simulink model "Model_V5"  (R2024b)
settings: Solver=VariableStepAuto  StartTime=0.0  StopTime=3600*12  RelTol=1e-3
undefined symbols (not defined in the file): PropsSI
libraries: fl_lib x569, SimscapeFluids_lib x61, nesl_utility x27
(part 2 of 7)

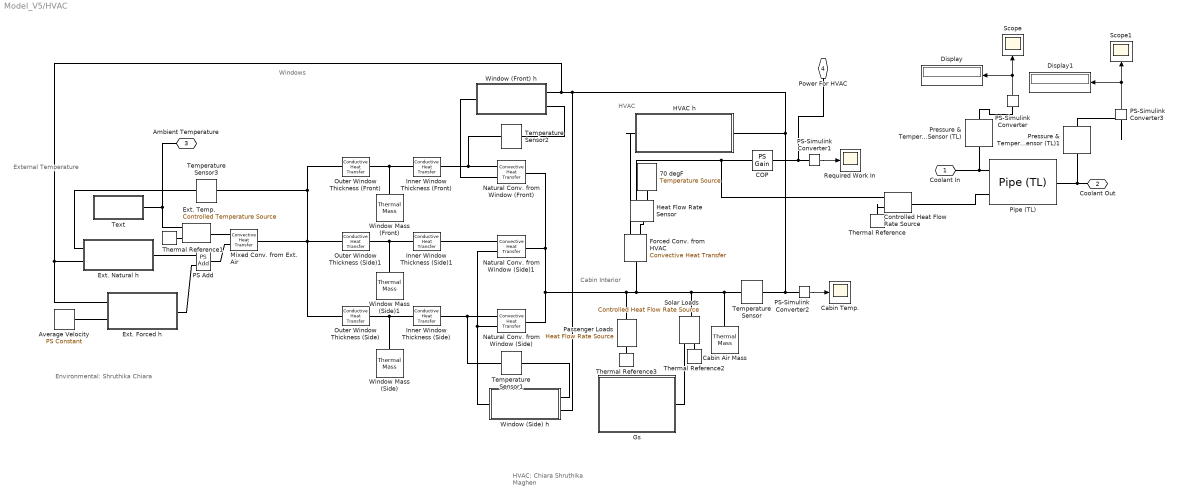
== system Model_V5/HVAC ==
  note: HVAC:
      | Chiara
      | Shruthika
      | Maghen
  note: Environmental:
      | Shruthika
      | Chiara
  note: Cabin Interior
  note: HVAC
  note: External Temperature
  note: Windows
  70 degF : fl_lib/Thermal/Thermal Sources/Temperature Source  temperature=70 degF
  Average Velocity : fl_lib/Physical Signals/Sources/PS Constant  constant=48 mi/hr
  COP : fl_lib/Physical Signals/Functions/PS Gain  gain=1/2
  Cabin Air Mass : fl_lib/Thermal/Thermal Elements/Thermal Mass  mass_type=foundation.enum.constant_variable.constant  mass=9.4009 kg  sp_heat=1005 J/(K*kg)  mass_min=1e-6 kg  num_ports=foundation.enum.numPorts2.one  m_specify=off  m_priority=High  m=1 kg  m_nominal_specify=off  m_nominal_value=1  m_nominal_unit=kg  T_specify=on  T_priority=Low  T=70 degF  T_nominal_specify=off  T_nominal_value=1  T_nominal_unit=K  Q_specify=off  Q_priority=None  Q=0 W  Q_nominal_specify=off  Q_nominal_value=1  Q_nominal_unit=W
  Cabin Temp. : Scope
  Controlled Heat Flow Rate Source : fl_lib/Thermal/Thermal Sources/Controlled Heat Flow Rate Source
  Display : Display
  Display1 : Display
  Ext. Forced h : Subsystem
  Ext. Natural h : Subsystem
  Ext. Temp. : fl_lib/Thermal/Thermal Sources/Controlled Temperature Source
  Forced Conv. from HVAC : fl_lib/Thermal/Thermal Elements/Convective Heat Transfer  thermal_type=foundation.enum.constant_variable.variable  area=19.0332 m^2  heat_tr_coeff=24.15 W/(K*m^2)  min_heat_tr_coeff=1e-3 W/(K*m^2)  T_specify=off  T_priority=None  T=0 K  T_nominal_specify=off  T_nominal_value=1  T_nominal_unit=K  Q_specify=off  Q_priority=None  Q=0 W  Q_nominal_specify=off  Q_nominal_value=1  Q_nominal_unit=W
      settings: InternalSimscapePortConfiguration="{\"Bottom\":[],\"Left\":[{\"id\":\"A\",\"label\":\"A\",\"type\":\"foundation.thermal.thermal\"},{\"id\":\"var_heat_tr_coeff\",\"label\":\"K\",\"type\":\"input\"}],\"Right\":[{\"id\":\"B\",\"label\":\"B\",\"type\":\"foundation.thermal.thermal\"}],\"Top\":[]}"
  Gs : Subsystem
  HVAC h : Subsystem
  Heat Flow Rate Sensor : fl_lib/Thermal/Thermal Sensors/Heat Flow Rate Sensor
  Inner Window Thickness (Front) : fl_lib/Thermal/Thermal Elements/Conductive Heat Transfer  thermal_type=foundation.enum.ConstantVariableTabulated.Constant  wall_geometry=foundation.enum.ConductionWallGeometry.Planar  area=40*55 in^2  thickness=0.25/2 in  d_in=0.05 m  d_out=0.1 m  L=1 m  th_cond_min=10 W/(K*m)  th_cond=1.05 W/(K*m)  th_cond_TLU=[413, 401, 392, 383, 371, 357, 342] W/(K*m)  temp_TLU=[200, 273, 400, 600, 800, 1000, 1200] K  T_specify=off  T_priority=None  T=0 K  T_nominal_specify=off  T_nominal_value=1  T_nominal_unit=K  Q_specify=off  Q_priority=None  Q=0 W  Q_nominal_specify=off  Q_nominal_value=1  Q_nominal_unit=W
  Inner Window Thickness (Side) : fl_lib/Thermal/Thermal Elements/Conductive Heat Transfer  thermal_type=foundation.enum.ConstantVariableTabulated.Constant  wall_geometry=foundation.enum.ConductionWallGeometry.Planar  area=40*40 in^2  thickness=0.25/2 in  d_in=0.05 m  d_out=0.1 m  L=1 m  th_cond_min=10 W/(K*m)  th_cond=1.05 W/(K*m)  th_cond_TLU=[413, 401, 392, 383, 371, 357, 342] W/(K*m)  temp_TLU=[200, 273, 400, 600, 800, 1000, 1200] K  T_specify=off  T_priority=None  T=0 K  T_nominal_specify=off  T_nominal_value=1  T_nominal_unit=K  Q_specify=off  Q_priority=None  Q=0 W  Q_nominal_specify=off  Q_nominal_value=1  Q_nominal_unit=W
  Inner Window Thickness (Side)1 : fl_lib/Thermal/Thermal Elements/Conductive Heat Transfer  thermal_type=foundation.enum.ConstantVariableTabulated.Constant  wall_geometry=foundation.enum.ConductionWallGeometry.Planar  area=40*40 in^2  thickness=0.25/2 in  d_in=0.05 m  d_out=0.1 m  L=1 m  th_cond_min=10 W/(K*m)  th_cond=1.05 W/(K*m)  th_cond_TLU=[413, 401, 392, 383, 371, 357, 342] W/(K*m)  temp_TLU=[200, 273, 400, 600, 800, 1000, 1200] K  T_specify=off  T_priority=None  T=0 K  T_nominal_specify=off  T_nominal_value=1  T_nominal_unit=K  Q_specify=off  Q_priority=None  Q=0 W  Q_nominal_specify=off  Q_nominal_value=1  Q_nominal_unit=W
  Mixed Conv. from Ext. Air : fl_lib/Thermal/Thermal Elements/Convective Heat Transfer  thermal_type=foundation.enum.constant_variable.variable  area=1e-4 m^2  heat_tr_coeff=20 W/(K*m^2)  min_heat_tr_coeff=1e-3 W/(K*m^2)  T_specify=off  T_priority=None  T=0 K  T_nominal_specify=off  T_nominal_value=1  T_nominal_unit=K  Q_specify=off  Q_priority=None  Q=0 W  Q_nominal_specify=off  Q_nominal_value=1  Q_nominal_unit=W
      settings: InternalSimscapePortConfiguration="{\"Bottom\":[],\"Left\":[{\"id\":\"A\",\"label\":\"A\",\"type\":\"foundation.thermal.thermal\"},{\"id\":\"var_heat_tr_coeff\",\"label\":\"K\",\"type\":\"input\"}],\"Right\":[{\"id\":\"B\",\"label\":\"B\",\"type\":\"foundation.thermal.thermal\"}],\"Top\":[]}"
  Natural Conv. from Window (Front) : fl_lib/Thermal/Thermal Elements/Convective Heat Transfer  thermal_type=foundation.enum.constant_variable.variable  area=1e-4 m^2  heat_tr_coeff=20 W/(K*m^2)  min_heat_tr_coeff=1e-3 W/(K*m^2)  T_specify=off  T_priority=None  T=0 K  T_nominal_specify=off  T_nominal_value=1  T_nominal_unit=K  Q_specify=off  Q_priority=None  Q=0 W  Q_nominal_specify=off  Q_nominal_value=1  Q_nominal_unit=W
      settings: InternalSimscapePortConfiguration="{\"Bottom\":[],\"Left\":[{\"id\":\"A\",\"label\":\"A\",\"type\":\"foundation.thermal.thermal\"},{\"id\":\"var_heat_tr_coeff\",\"label\":\"K\",\"type\":\"input\"}],\"Right\":[{\"id\":\"B\",\"label\":\"B\",\"type\":\"foundation.thermal.thermal\"}],\"Top\":[]}"
  Natural Conv. from Window (Side) : fl_lib/Thermal/Thermal Elements/Convective Heat Transfer  thermal_type=foundation.enum.constant_variable.variable  area=1e-4 m^2  heat_tr_coeff=20 W/(K*m^2)  min_heat_tr_coeff=1e-3 W/(K*m^2)  T_specify=off  T_priority=None  T=0 K  T_nominal_specify=off  T_nominal_value=1  T_nominal_unit=K  Q_specify=off  Q_priority=None  Q=0 W  Q_nominal_specify=off  Q_nominal_value=1  Q_nominal_unit=W
      settings: InternalSimscapePortConfiguration="{\"Bottom\":[],\"Left\":[{\"id\":\"A\",\"label\":\"A\",\"type\":\"foundation.thermal.thermal\"},{\"id\":\"var_heat_tr_coeff\",\"label\":\"K\",\"type\":\"input\"}],\"Right\":[{\"id\":\"B\",\"label\":\"B\",\"type\":\"foundation.thermal.thermal\"}],\"Top\":[]}"
  Natural Conv. from Window (Side)1 : fl_lib/Thermal/Thermal Elements/Convective Heat Transfer  thermal_type=foundation.enum.constant_variable.variable  area=1e-4 m^2  heat_tr_coeff=20 W/(K*m^2)  min_heat_tr_coeff=1e-3 W/(K*m^2)  T_specify=off  T_priority=None  T=0 K  T_nominal_specify=off  T_nominal_value=1  T_nominal_unit=K  Q_specify=off  Q_priority=None  Q=0 W  Q_nominal_specify=off  Q_nominal_value=1  Q_nominal_unit=W
      settings: InternalSimscapePortConfiguration="{\"Bottom\":[],\"Left\":[{\"id\":\"A\",\"label\":\"A\",\"type\":\"foundation.thermal.thermal\"},{\"id\":\"var_heat_tr_coeff\",\"label\":\"K\",\"type\":\"input\"}],\"Right\":[{\"id\":\"B\",\"label\":\"B\",\"type\":\"foundation.thermal.thermal\"}],\"Top\":[]}"
  Outer Window Thickness (Front) : fl_lib/Thermal/Thermal Elements/Conductive Heat Transfer  thermal_type=foundation.enum.ConstantVariableTabulated.Constant  wall_geometry=foundation.enum.ConductionWallGeometry.Planar  area=40*55 in^2  thickness=0.25/2 m  d_in=0.05 m  d_out=0.1 m  L=1 m  th_cond_min=10 W/(K*m)  th_cond=1.05 W/(K*m)  th_cond_TLU=[413, 401, 392, 383, 371, 357, 342] W/(K*m)  temp_TLU=[200, 273, 400, 600, 800, 1000, 1200] K  T_specify=off  T_priority=None  T=0 K  T_nominal_specify=off  T_nominal_value=1  T_nominal_unit=K  Q_specify=off  Q_priority=None  Q=0 W  Q_nominal_specify=off  Q_nominal_value=1  Q_nominal_unit=W
  Outer Window Thickness (Side) : fl_lib/Thermal/Thermal Elements/Conductive Heat Transfer  thermal_type=foundation.enum.ConstantVariableTabulated.Constant  wall_geometry=foundation.enum.ConductionWallGeometry.Planar  area=40*40 in^2  thickness=0.25/2 m  d_in=0.05 m  d_out=0.1 m  L=1 m  th_cond_min=10 W/(K*m)  th_cond=1.05 W/(K*m)  th_cond_TLU=[413, 401, 392, 383, 371, 357, 342] W/(K*m)  temp_TLU=[200, 273, 400, 600, 800, 1000, 1200] K  T_specify=off  T_priority=None  T=0 K  T_nominal_specify=off  T_nominal_value=1  T_nominal_unit=K  Q_specify=off  Q_priority=None  Q=0 W  Q_nominal_specify=off  Q_nominal_value=1  Q_nominal_unit=W
  Outer Window Thickness (Side)1 : fl_lib/Thermal/Thermal Elements/Conductive Heat Transfer  thermal_type=foundation.enum.ConstantVariableTabulated.Constant  wall_geometry=foundation.enum.ConductionWallGeometry.Planar  area=40*40 in^2  thickness=0.25/2 m  d_in=0.05 m  d_out=0.1 m  L=1 m  th_cond_min=10 W/(K*m)  th_cond=1.05 W/(K*m)  th_cond_TLU=[413, 401, 392, 383, 371, 357, 342] W/(K*m)  temp_TLU=[200, 273, 400, 600, 800, 1000, 1200] K  T_specify=off  T_priority=None  T=0 K  T_nominal_specify=off  T_nominal_value=1  T_nominal_unit=K  Q_specify=off  Q_priority=None  Q=0 W  Q_nominal_specify=off  Q_nominal_value=1  Q_nominal_unit=W
  PS Add : fl_lib/Physical Signals/Functions/PS Add
  PS-Simulink Converter : nesl_utility/PS-Simulink Converter  PhysicalDomain=network_engine_domain  SubClassName=ps_output  LeftPortType=input  RightPortType=output  PseudoPeriodic=off  Frequencies=[]  VectorFormat=inherit  Unit=degF  AffineConversion=on
  PS-Simulink Converter1 : nesl_utility/PS-Simulink Converter  PhysicalDomain=network_engine_domain  SubClassName=ps_output  LeftPortType=input  RightPortType=output  PseudoPeriodic=off  Frequencies=[]  VectorFormat=inherit  Unit=inherit  AffineConversion=off
  PS-Simulink Converter2 : nesl_utility/PS-Simulink Converter  PhysicalDomain=network_engine_domain  SubClassName=ps_output  LeftPortType=input  RightPortType=output  PseudoPeriodic=off  Frequencies=[]  VectorFormat=inherit  Unit=degF  AffineConversion=on
  PS-Simulink Converter3 : nesl_utility/PS-Simulink Converter  PhysicalDomain=network_engine_domain  SubClassName=ps_output  LeftPortType=input  RightPortType=output  PseudoPeriodic=off  Frequencies=[]  VectorFormat=inherit  Unit=degF  AffineConversion=on
  Passenger Loads : fl_lib/Thermal/Thermal Sources/Heat Flow Rate Source  heat_flow=6*104 W
      settings: InternalSimscapePortConfiguration="{\"Bottom\":[],\"Left\":[{\"id\":\"B\",\"label\":\"B\",\"type\":\"foundation.thermal.thermal\"}],\"Right\":[{\"id\":\"A\",\"label\":\"A\",\"type\":\"foundation.thermal.thermal\"}],\"Top\":[]}"
  Pipe (TL) : SimscapeFluids_lib/Thermal Liquid/Pipes & Fittings/Pipe (TL)  dynamic_compressibility=true  inertia=false  num_segments=1  pipe_length=5 m  cross_section_geometry=fluids.thermal_liquid.pipes_fittings.enum.CrossSectionGeometry.Circular  pipe_diameter=1.5 in  pipe_inner_diameter=0.05 m  pipe_outer_diameter=0.1 m  pipe_width=0.1 m  pipe_height=0.1 m  pipe_major_axis=0.1 m  pipe_minor_axis=0.05 m  pipe_side=0.1 m  pipe_angle=30 deg  area=0.01 m^2  Dh=0.1128 m  elevation_spec=foundation.enum.constant_variable.constant  elevation_gain=0 m  gravity_spec=foundation.enum.constant_variable.constant  g=9.81 m/s^2  pressure_loss_spec=fluids.thermal_liquid.pipes_fittings.enum.PressureLossSpec.Haaland  local_pressure_loss_spec=fluids.thermal_liquid.pipes_fittings.enum.LocalLossSpec.AggregateLength  length_add=1 m  loss_coefficient=0.1  roughness_spec=fluids.thermal_liquid.pipes_fittings.enum.RoughnessSpec.CommercialPipe  roughness=15e-6 m  Re_friction_TLU=[400, 1000, 1500, 3000, 4000, 6000, 10000, 20000, 40000, 60000, 100000, 100000000]  friction_factor_TLU=[.264, .112, .071, .0417, .0387, .0268, .025, .0232, .0226, .022, .0214, .0214]  Re_lam=2000  Re_tur=4000  shape_factor=64  mdot_nominal=[.1, 1] kg/s  p_diff_nominal=[.001, .01] MPa  mdot_threshold=1e-6 kg/s  wall_spec=fluids.thermal_liquid.pipes_fittings.enum.wall_spec.rigid  vol_expansion_spec=fluids.thermal_liquid.pipes_fittings.enum.VolumeExpansionSpec.Area  area_pressure_gain=1e-6 m^2/MPa  static_pressure_TLU=[.1, 1] MPa  area_pressure_gain_TLU=[1e-05, 1.1e-05] m^2  material_behavior_spec=fluids.thermal_liquid.pipes_fittings.enum.PipeMaterialBehavior.Linear  diameter_pressure_gain=1e-6 m/MPa  wall_thickness=0.05 m  elastic_modulus=69 GPa  stress_TLU=[276, 310] MPa  strain_TLU=[.004, .02]  stress_assert_action=simscape.enum.assert.action.none  stress_max=400 MPa  poisson_ratio=0.33  wall_time_constant=0.01 s  thermal_expansion=false  alpha_L_wall=24 um/(deltaK*m)  thermal_expansion_Tref=293.15 K  heat_transfer_spec=fluids.thermal_liquid.pipes_fittings.enum.HeatTransferSpec.Gnielinski  mdot_nominal_heat=[.1, 1] kg/s  T_in_nominal=[293.15, 293.15] K  T_out_nominal=[300, 300] K  p_in_nominal_heat=[.101325, .101325] MPa  T_wall_nominal=[303.15, 303.15] K  a_coeff=0.023  b_Re_power=0.8  c_Pr_power=0.4  Nu_lam=3.66  Re_Colburn_TLU=[100, 150, 1000]  Colburn_factor_TLU=[.019, .013, .002]  Re_Nu_TLU=[100, 150, 1000]  Pr_Nu_TLU=[1, 10]  Nu_TLU=[3.72, 4.21; 3.75, 4.44; 4.21, 7.15]  p0_vec=0.101325 MPa  T0_vec=293.15 K  mdot0=0.1 kg/s
  Pressure & Temperature Sensor (TL) : fl_lib/Thermal Liquid/Sensors/Pressure & Temperature Sensor (TL)  reference=foundation.enum.MeasurementReference.absolute  pressure=false  pressure_spec=foundation.enum.PressureMeasementSpec.Absolute  temperature=true
      settings: InternalSimscapePortConfiguration="{\"Bottom\":[{\"id\":\"T\",\"label\":\"T\",\"type\":\"output\"}],\"Left\":[{\"id\":\"A\",\"label\":\"A\",\"type\":\"foundation.thermal_liquid.thermal_liquid\"}],\"Right\":[],\"Top\":[]}"
  Pressure & Temperature Sensor (TL)1 : fl_lib/Thermal Liquid/Sensors/Pressure & Temperature Sensor (TL)  reference=foundation.enum.MeasurementReference.absolute  pressure=false  pressure_spec=foundation.enum.PressureMeasementSpec.Absolute  temperature=true
      settings: InternalSimscapePortConfiguration="{\"Bottom\":[{\"id\":\"T\",\"label\":\"T\",\"type\":\"output\"}],\"Left\":[{\"id\":\"A\",\"label\":\"A\",\"type\":\"foundation.thermal_liquid.thermal_liquid\"}],\"Right\":[],\"Top\":[]}"
  Required Work In : Scope
  Scope : Scope
  Scope1 : Scope
  Solar Loads : fl_lib/Thermal/Thermal Sources/Controlled Heat Flow Rate Source
  Temperature Sensor{,1..3} (4 alike) : fl_lib/Thermal/Thermal Sensors/Temperature Sensor  temperature_measure=foundation.enum.MeasurementReference.absolute
      settings: InternalSimscapePortConfiguration="{\"Bottom\":[],\"Left\":[{\"id\":\"A\",\"label\":\"A\",\"type\":\"foundation.thermal.thermal\"}],\"Right\":[{\"id\":\"T\",\"label\":\"T\",\"type\":\"output\"}],\"Top\":[]}"
  Text : Subsystem
  Thermal Reference{,1..3} (4 alike) : fl_lib/Thermal/Thermal Elements/Thermal Reference
  Window (Front) h : Subsystem
  Window (Side) h : Subsystem
  Window Mass (Front) : fl_lib/Thermal/Thermal Elements/Thermal Mass  mass_type=foundation.enum.constant_variable.constant  mass=23.2442 kg  sp_heat=840 J/(K*kg)  mass_min=1e-6 kg  num_ports=foundation.enum.numPorts2.one  m_specify=off  m_priority=High  m=1 kg  m_nominal_specify=off  m_nominal_value=1  m_nominal_unit=kg  T_specify=on  T_priority=Low  T=70 degF  T_nominal_specify=off  T_nominal_value=1  T_nominal_unit=K  Q_specify=off  Q_priority=None  Q=0 W  Q_nominal_specify=off  Q_nominal_value=1  Q_nominal_unit=W
  Window Mass (Side) : fl_lib/Thermal/Thermal Elements/Thermal Mass  mass_type=foundation.enum.constant_variable.constant  mass=16.9049 kg  sp_heat=840 J/(K*kg)  mass_min=1e-6 kg  num_ports=foundation.enum.numPorts2.one  m_specify=off  m_priority=High  m=1 kg  m_nominal_specify=off  m_nominal_value=1  m_nominal_unit=kg  T_specify=on  T_priority=Low  T=70 degF  T_nominal_specify=off  T_nominal_value=1  T_nominal_unit=K  Q_specify=off  Q_priority=None  Q=0 W  Q_nominal_specify=off  Q_nominal_value=1  Q_nominal_unit=W
  Window Mass (Side)1 : fl_lib/Thermal/Thermal Elements/Thermal Mass  mass_type=foundation.enum.constant_variable.constant  mass=16.9049 kg  sp_heat=840 J/(K*kg)  mass_min=1e-6 kg  num_ports=foundation.enum.numPorts2.one  m_specify=off  m_priority=High  m=1 kg  m_nominal_specify=off  m_nominal_value=1  m_nominal_unit=kg  T_specify=on  T_priority=Low  T=70 degF  T_nominal_specify=off  T_nominal_value=1  T_nominal_unit=K  Q_specify=off  Q_priority=None  Q=0 W  Q_nominal_specify=off  Q_nominal_value=1  Q_nominal_unit=W
  Coolant In : PMIOPort  Side=Left
  Coolant Out : PMIOPort  Port=2  Side=Left
  Ambient Temperature : PMIOPort  Port=3  Side=Right
  Power For HVAC : PMIOPort  Port=4  Side=Right
  wires:
  PS-Simulink Converter1/1 -> Required Work In/1
  PS-Simulink Converter2/1 -> Cabin Temp./1
  PS-Simulink Converter/1 -> Display/1, Scope/1
  PS-Simulink Converter3/1 -> Scope1/1, Display1/1
  connections:
  Inner Window Thickness (Side)/LConn1 -- Outer Window Thickness (Side)/RConn1 -- Window Mass (Side)/LConn1
  Window Mass (Side)1/LConn1 -- Inner Window Thickness (Side)1/LConn1 -- Outer Window Thickness (Side)1/RConn1
  Temperature Sensor/RConn1 -- PS-Simulink Converter2/LConn1 -- HVAC h/LConn1 -- Ext. Forced h/LConn1 -- Ext. Natural h/LConn2 -- Window (Front) h/LConn1 -- Window (Side) h/LConn2
  Outer Window Thickness (Front)/RConn1 -- Inner Window Thickness (Front)/LConn1 -- Window Mass (Front)/LConn1
  Natural Conv. from Window (Side)/LConn1 -- Temperature Sensor1/LConn1 -- Inner Window Thickness (Side)/RConn1
  Outer Window Thickness (Front)/LConn1 -- Temperature Sensor3/LConn1 -- Mixed Conv. from Ext. Air/RConn1 -- Outer Window Thickness (Side)1/LConn1 -- Outer Window Thickness (Side)/LConn1
  Heat Flow Rate Sensor/RConn2 -- 70 degF/LConn1
  Passenger Loads/LConn1 -- Solar Loads/LConn1 -- Temperature Sensor/LConn1 -- Cabin Air Mass/LConn1 -- Forced Conv. from HVAC/RConn1 -- Natural Conv. from Window (Side)/RConn1 -- Natural Conv. from Window (Front)/RConn1 -- Natural Conv. from Window (Side)1/RConn1
  Inner Window Thickness (Front)/RConn1 -- Natural Conv. from Window (Front)/LConn1 -- Temperature Sensor2/LConn1
  Window (Side) h/RConn1 -- Natural Conv. from Window (Side)1/LConn2 -- Natural Conv. from Window (Side)/LConn2
  Temperature Sensor3/RConn1 -- Ext. Natural h/LConn1
  Natural Conv. from Window (Side)1/LConn1 -- Inner Window Thickness (Side)1/RConn1
  Text/RConn1 -- Ext. Temp./RConn1 -- Ambient Temperature/RConn1
  Average Velocity/RConn1 -- Ext. Forced h/LConn2
  Ext. Forced h/RConn1 -- PS Add/LConn2
  Temperature Sensor1/RConn1 -- Window (Side) h/LConn1
  Coolant Out/RConn1 -- Pressure & Temperature Sensor (TL)1/LConn1 -- Pipe (TL)/RConn1
  Ext. Natural h/RConn1 -- PS Add/LConn1
  Thermal Reference3/LConn1 -- Passenger Loads/RConn1
  PS Add/RConn1 -- Mixed Conv. from Ext. Air/LConn2
  Coolant In/RConn1 -- Pressure & Temperature Sensor (TL)/LConn1 -- Pipe (TL)/LConn1
  PS-Simulink Converter1/LConn1 -- COP/RConn1 -- Power For HVAC/RConn1
  Thermal Reference1/LConn1 -- Ext. Temp./RConn2
  HVAC h/RConn1 -- Forced Conv. from HVAC/LConn2
  COP/LConn1 -- Controlled Heat Flow Rate Source/RConn1 -- Heat Flow Rate Sensor/RConn1
  Solar Loads/RConn2 -- Thermal Reference2/LConn1
  Mixed Conv. from Ext. Air/LConn1 -- Ext. Temp./LConn1
  Gs/RConn1 -- Solar Loads/RConn1
  Temperature Sensor2/RConn1 -- Window (Front) h/LConn2
  Window (Front) h/RConn1 -- Natural Conv. from Window (Front)/LConn2
  Forced Conv. from HVAC/LConn1 -- Heat Flow Rate Sensor/LConn1
  Pressure & Temperature Sensor (TL)/RConn1 -- PS-Simulink Converter/LConn1
  PS-Simulink Converter3/LConn1 -- Pressure & Temperature Sensor (TL)1/RConn1
  Controlled Heat Flow Rate Source/LConn1 -- Pipe (TL)/LConn2
  Thermal Reference/LConn1 -- Controlled Heat Flow Rate Source/RConn2

== system Model_V5/Inverter ==
  note: Inverter:
      | Bella
  note: TIM is silver paste
      | (STCH)
  note: Rjb is set to infinity so that
      | the design is based off all the
      | heat flowing soley to the cold plate.
      | A realistic Rjb value would benefit
      | heat dissipation.
      | TJmax = 125degC
  note: Inlet coolant temp 50degC or below
  Battery Loss : fl_lib/Physical Signals/Functions/PS Gain  gain=0.9
  Display : Display
  Dividing it for 4 inverters : fl_lib/Physical Signals/Functions/PS Gain  gain=1/4
  Efficiency Subsystem : Subsystem
  Elbow (TL){,1..3} (4 alike) : SimscapeFluids_lib/Thermal Liquid/Pipes & Fittings/Elbow (TL)  elbow_type=fluids.thermal_liquid.pipes_fittings.enum.ElbowType.Smooth  diameter_elbow=1.5 in  angle_elbow=90 deg  Re_c=150
      settings: InternalSimscapePortConfiguration="{\"Bottom\":[],\"Left\":[{\"id\":\"A\",\"label\":\"A\",\"type\":\"foundation.thermal_liquid.thermal_liquid\"}],\"Right\":[],\"Top\":[{\"id\":\"B\",\"label\":\"B\",\"type\":\"foundation.thermal_liquid.thermal_liquid\"}]}"
  Inverter 1 : Subsystem
  Inverter 2 : Subsystem
  Inverter 3 : Subsystem
  Inverter 4 : Subsystem
  PS Constant : fl_lib/Physical Signals/Sources/PS Constant  constant=0.9
  PS-Simulink Converter : nesl_utility/PS-Simulink Converter  PhysicalDomain=network_engine_domain  SubClassName=ps_output  LeftPortType=input  RightPortType=output  PseudoPeriodic=off  Frequencies=[]  VectorFormat=inherit  Unit=degC  AffineConversion=on
  PS-Simulink Converter6 : nesl_utility/PS-Simulink Converter  PhysicalDomain=network_engine_domain  SubClassName=ps_output  LeftPortType=input  RightPortType=output  PseudoPeriodic=off  Frequencies=[]  VectorFormat=inherit  Unit=degC  AffineConversion=on
  Pressure & Temperature Sensor (TL)1 : fl_lib/Thermal Liquid/Sensors/Pressure & Temperature Sensor (TL)  reference=foundation.enum.MeasurementReference.absolute  pressure=false  pressure_spec=foundation.enum.PressureMeasementSpec.Absolute  temperature=true
      settings: InternalSimscapePortConfiguration="{\"Bottom\":[{\"id\":\"T\",\"label\":\"T\",\"type\":\"output\"}],\"Left\":[{\"id\":\"A\",\"label\":\"A\",\"type\":\"foundation.thermal_liquid.thermal_liquid\"}],\"Right\":[],\"Top\":[]}"
  Scope6 : Scope
  T-Junction (TL){,1..5} (6 alike) : SimscapeFluids_lib/Thermal Liquid/Pipes & Fittings/T-Junction (TL)  area_main=0.0011 m^2  area_branch=0.0011 m^2  junction_spec=fluids.thermal_liquid.pipes_fittings.enum.TLossCoefficientModel.Crane  k_main_converge=1.12  k_main_diverge=1.12  k_branch_converge=1.12  k_branch_diverge=1.12  loss_coeff_A=1  loss_coeff_B=1  loss_coeff_C=1  radius=0.001 m  Re_c=150  Re_0=10  tau=0.0001 s  saturation_ratio=0.2  smoothing_factor=0.01  inertia=false
      settings: InternalSimscapePortConfiguration="{\"Bottom\":[{\"id\":\"C\",\"label\":\"C\",\"type\":\"foundation.thermal_liquid.thermal_liquid\"}],\"Left\":[{\"id\":\"A\",\"label\":\"A\",\"type\":\"foundation.thermal_liquid.thermal_liquid\"}],\"Right\":[{\"id\":\"B\",\"label\":\"B\",\"type\":\"foundation.thermal_liquid.thermal_liquid\"}],\"Top\":[]}"
  Temperature Sensor : fl_lib/Thermal/Thermal Sensors/Temperature Sensor  temperature_measure=foundation.enum.MeasurementReference.absolute
      settings: InternalSimscapePortConfiguration="{\"Bottom\":[],\"Left\":[{\"id\":\"A\",\"label\":\"A\",\"type\":\"foundation.thermal.thermal\"}],\"Right\":[{\"id\":\"T\",\"label\":\"T\",\"type\":\"output\"}],\"Top\":[]}"
  Power In : PMIOPort  Side=Left
  Coolant In : PMIOPort  Port=2  Side=Right
  Coolant Out : PMIOPort  Port=3  Side=Right
  Coolant Inlet Temp : Outport
  IGBT Temp : Outport  Port=2
  wires:
  PS-Simulink Converter6/1 -> Coolant Inlet Temp/1, Scope6/1, Display/1
  PS-Simulink Converter/1 -> IGBT Temp/1
  connections:
  PS Constant/RConn1 -- Efficiency Subsystem/LConn1
  Battery Loss/LConn1 -- Power In/RConn1
  Battery Loss/RConn1 -- Efficiency Subsystem/LConn2
  Dividing it for 4 inverters/LConn1 -- Efficiency Subsystem/RConn1
  PS-Simulink Converter6/LConn1 -- Pressure & Temperature Sensor (TL)1/RConn1
  PS-Simulink Converter/LConn1 -- Temperature Sensor/RConn1
  Coolant In/RConn1 -- Pressure & Temperature Sensor (TL)1/LConn1 -- T-Junction (TL)/RConn2
  Temperature Sensor/LConn1 -- Inverter 4/RConn1
  Inverter 1/LConn2 -- Inverter 4/LConn2 -- Inverter 3/LConn2 -- Inverter 2/LConn2 -- Dividing it for 4 inverters/RConn1
  T-Junction (TL)1/LConn1 -- T-Junction (TL)/LConn1
  Elbow (TL)1/LConn1 -- T-Junction (TL)2/LConn1
  T-Junction (TL)2/RConn1 -- T-Junction (TL)/RConn1
  Elbow (TL)/LConn2 -- T-Junction (TL)1/RConn1
  Elbow (TL)/LConn1 -- Inverter 4/LConn1
  T-Junction (TL)1/RConn2 -- Inverter 3/LConn1
  T-Junction (TL)2/RConn2 -- Inverter 2/LConn1
  Elbow (TL)1/LConn2 -- Inverter 1/LConn1
  Elbow (TL)2/LConn2 -- Inverter 4/RConn2
  T-Junction (TL)3/RConn2 -- Inverter 3/RConn1
  T-Junction (TL)3/LConn1 -- Elbow (TL)2/LConn1
  T-Junction (TL)4/RConn2 -- Inverter 2/RConn1
  T-Junction (TL)5/RConn1 -- T-Junction (TL)3/RConn1
  T-Junction (TL)5/LConn1 -- T-Junction (TL)4/LConn1
  T-Junction (TL)5/RConn2 -- Coolant Out/RConn1
  Elbow (TL)3/LConn1 -- Inverter 1/RConn1
  Elbow (TL)3/LConn2 -- T-Junction (TL)4/RConn1
